simulink model "AMCLIB_TrackObsrv_BAM_FLT"  (Simulink 8.3)
settings: Solver=ode45  StartTime=0.0  StopTime=10.0  RelTol=1e-3
undefined symbols (not defined in the file): fltC1, fltCC1, fltCC2
settings Model: Creator=RE004C  LastModifiedBy=RE004C
settings DataIOCC: SignalLoggingSaveFormat=Dataset
settings DebuggingCC: UnderspecifiedInitializationDetection=Simplified  StateNameClashWarn=none
settings GRTTargetCC: CombineOutputUpdateFcns=on  GRTInterface=off

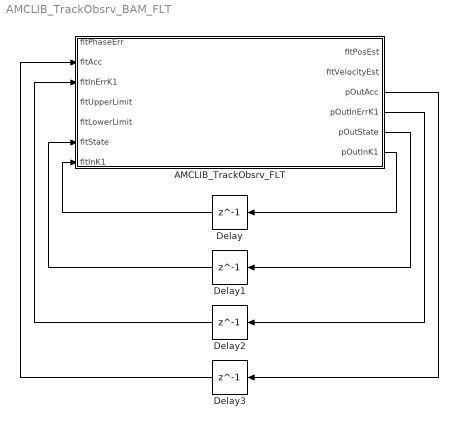
== system AMCLIB_TrackObsrv_BAM_FLT ==
  AMCLIB_TrackObsrv_FLT : Subsystem  mask(AMCLIB_TrackObsrv_FLT){fltCC1=fltCC1, fltCC2=fltCC2, fltC1=fltC1}
      mask help: Bit accurate model of the tracking observer function.
      mask init:
      | pos = get_param(gcb, 'Position');width = pos(3) - pos(1); height = pos(4) - pos(2);tX=width/2;tY=height*0.9;
      mask Display: color('black');port_label('input',1,'fltPhaseErr');port_label('input',2,'fltAcc');port_label('input',3,'fltInErrK1');port_label('input',4,'fltUpperLimit');port_label('input',5,'fltLowerLimit');port_label('input',6,'fltState');port_label('input',7,'fltInK1');port_label('output',1,'fltPosEst');port_label('output',2,'fltVelocityEst');port_label('output',3,'pOutAcc');port_label('output',4,'pOutInErrK1');port_label('output',5,'pOutState');port_label('output',6,'pOutInK1');color('black');disp('AMCLIB_TrackObsrv_FLT');color('blue');text(tX,tY, 'BAM', 'horizontalAlignment', 'center');
  Delay{,1..3} (4 alike) : Delay  DelayLength=1  InitialCondition=0
  wires:
  AMCLIB_TrackObsrv_FLT/6(pOutInK1) -> Delay/1
  AMCLIB_TrackObsrv_FLT/5(pOutState) -> Delay1/1
  AMCLIB_TrackObsrv_FLT/4(pOutInErrK1) -> Delay2/1
  AMCLIB_TrackObsrv_FLT/3(pOutAcc) -> Delay3/1
  Delay/1 -> AMCLIB_TrackObsrv_FLT/7(fltInK1)
  Delay1/1 -> AMCLIB_TrackObsrv_FLT/6(fltState)
  Delay2/1 -> AMCLIB_TrackObsrv_FLT/3(fltInErrK1)
  Delay3/1 -> AMCLIB_TrackObsrv_FLT/2(fltAcc)

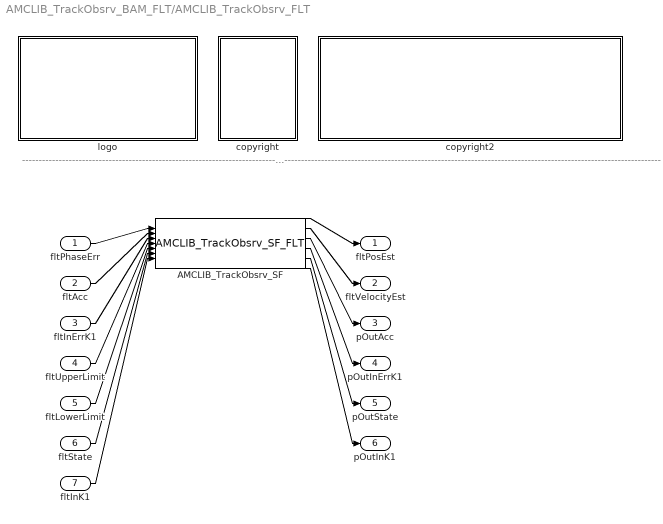
== system AMCLIB_TrackObsrv_BAM_FLT/AMCLIB_TrackObsrv_FLT ==
  note: ---------------------------------------------------------------------------------------------------------------------------------------------------------------------------------------------------
  fltPhaseErr : Inport
  fltAcc : Inport  Port=2
  fltInErrK1 : Inport  Port=3
  fltUpperLimit : Inport  Port=4
  fltLowerLimit : Inport  Port=5
  fltState : Inport  Port=6
  fltInK1 : Inport  Port=7
  AMCLIB_TrackObsrv_SF : S-Function  FunctionName=AMCLIB_TrackObsrv_SF_FLT  Parameters=fltCC1,fltCC2,fltC1  EnableBusSupport=off
  copyright : Subsystem
      mask Display: text(10,90,'FILE:');text(10,75,'DESRIPTION:');text(10,60,'COPYRIGHT:');text(10,45,'VERSION:');text(10,30,'DATE:')
  copyright2 : Subsystem
      mask Display: text(10,90,'AMCLIB_TrackObsrv_BAM_FLT.mdl');text(10,75,'Tracking observer function.');text(10,60,'NXP');text(10,45,'1.0');text(10,30,'29-Jul-2016');
  logo : Subsystem
      mask Display: image(imread('logo.jpg'))
  fltPosEst : Outport
  fltVelocityEst : Outport  Port=2
  pOutAcc : Outport  Port=3
  pOutInErrK1 : Outport  Port=4
  pOutState : Outport  Port=5
  pOutInK1 : Outport  Port=6
  wires:
  fltPhaseErr/1 -> AMCLIB_TrackObsrv_SF/1
  fltAcc/1 -> AMCLIB_TrackObsrv_SF/2
  fltInErrK1/1 -> AMCLIB_TrackObsrv_SF/3
  fltUpperLimit/1 -> AMCLIB_TrackObsrv_SF/4
  fltLowerLimit/1 -> AMCLIB_TrackObsrv_SF/5
  fltState/1 -> AMCLIB_TrackObsrv_SF/6
  fltInK1/1 -> AMCLIB_TrackObsrv_SF/7
  AMCLIB_TrackObsrv_SF/1 -> fltPosEst/1
  AMCLIB_TrackObsrv_SF/2 -> fltVelocityEst/1
  AMCLIB_TrackObsrv_SF/3 -> pOutAcc/1
  AMCLIB_TrackObsrv_SF/4 -> pOutInErrK1/1
  AMCLIB_TrackObsrv_SF/5 -> pOutState/1
  AMCLIB_TrackObsrv_SF/6 -> pOutInK1/1

== system AMCLIB_TrackObsrv_BAM_FLT/AMCLIB_TrackObsrv_FLT/copyright ==

== system AMCLIB_TrackObsrv_BAM_FLT/AMCLIB_TrackObsrv_FLT/copyright2 ==

== system AMCLIB_TrackObsrv_BAM_FLT/AMCLIB_TrackObsrv_FLT/logo ==
